simulink model "test_model_2"  (R2017a)
settings: Solver=VariableStepAuto  StartTime=0.0  StopTime=inf  RelTol=1e-3
undefined symbols (not defined in the file): AUV, HydroDyn, kc, Z_delay
libraries: slrealtimeutilitieslib x2, slrealtimeiplib x2, sldrtlib x1, simulink x1
settings Model: Creator=117-11  LastModifiedBy=corsair
settings SFSimCC: SimUseLocalCustomCode=on
settings RTWCC: RTWUseLocalCustomCode=on

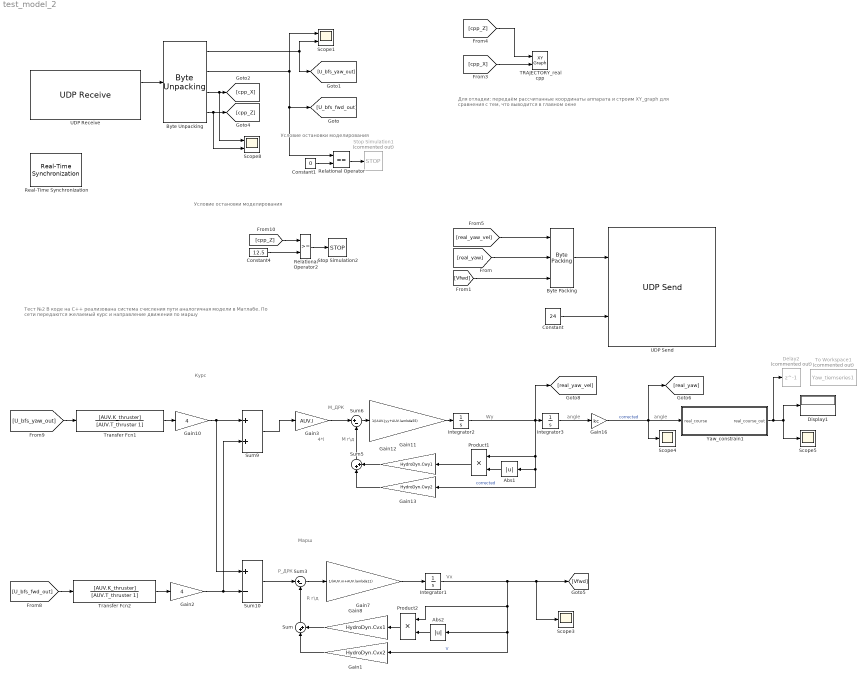
== system test_model_2 ==
  note: Тест №2
      |
      | В коде на С++ реализована система счисления пути аналогичная модели в Матлабе.
      | По сети передаются желаемый курс и направление движения по маршу
  note: Условие остановки моделирования
  note: Для отладки: передаём рассчитанные координаты аппарата и строим XY_graph для сравнения с тем, что выводится в главном окне
  note: Курс
  note: 4*l
  note: Марш
  note: angle
  note: R г\д
  note: Wy
  note: P_ДРК
  note: M_ДРК
  note: M г\д
  note: Vx
  note: angle
  note: Условие остановки моделирования
  Abs1 : Abs
  Abs2 : Abs
  "Byte Packing " : slrealtimeutilitieslib/Byte Packing  MaskPackedDataType=uint8  MaskUnpackedDataTypes={'double', 'double', 'double'}  MaskAlignment=1
  "Byte Unpacking " : slrealtimeutilitieslib/Byte Unpacking  MaskUnpackedDataTypes={'double', 'double', 'double', 'double'}  MaskUnpackedDataSizes={[1], [1], [1], [1]}  MaskAlignment=1
      settings: SourceProductBaseCode=XP
  Constant : Constant  Value=24
  Constant1 : Constant  Value=0
  Constant4 : Constant  Value=12.5
  Delay2 : Delay  Commented=on  DelayLength=1  InitialCondition=180  SampleTime=Z_delay
  Display1 : Display
  Gain1 : Gain  Gain=HydroDyn.Cvx2
  Gain10 : Gain  Gain=4
  Gain11 : Gain  Gain=1/(AUV.Jyy+AUV.lambda55)
  Gain12 : Gain  Gain=HydroDyn.Cwy1
  Gain13 : Gain  Gain=HydroDyn.Cwy2
  Gain16 : Gain  Gain=kc
  Gain2 : Gain  Gain=4
  Gain3 : Gain  Gain=AUV.l
  Gain7 : Gain  Gain=1/(AUV.m+AUV.lambda11)
  Gain8 : Gain  Gain=HydroDyn.Cvx1
  Integrator1 : Integrator  InitialCondition=0.7
  Integrator2 : Integrator
  Integrator3 : Integrator  InitialCondition=3.1416
  Product1 : Product
  Product2 : Product
  Real-Time Synchronization : sldrtlib/Real-Time Synchronization  SampleTime=0.001  MaxMissedTicks=10  ShowMissedTicks=off  YieldWhenWaiting=off
  Relational Operator : RelationalOperator  Operator===  OutDataTypeStr=boolean  RndMeth=Simplest
  Relational Operator2 : RelationalOperator  OutDataTypeStr=boolean  RndMeth=Simplest
  Scope1 : Scope  NumInputPorts=2
  Scope3 : Scope
  Scope4 : Scope
  Scope5 : Scope
  Scope8 : Scope  NumInputPorts=2
  Stop Simulation1 : Stop  Commented=on
  Stop Simulation2 : Stop
  Sum : Sum  Inputs=|++
  Sum10 : Sum  Inputs=+-
  Sum3 : Sum  Inputs=|+-
  Sum5 : Sum  Inputs=|++
  Sum6 : Sum  Inputs=|+-
  Sum9 : Sum
  TRAJECTORY_real cpp : simulink/Sinks/XY Graph  xmin=-15  xmax=15  ymin=-15  ymax=15  st=Z_delay
  To Workspace1 : ToWorkspace  Commented=on  VariableName=Yaw_tiemseries1  SaveFormat=Timeseries  SampleTime=-1
  Transfer Fcn1 : TransferFcn  Numerator=[AUV.K_thruster]  Denominator=[AUV.T_thruster 1]
  Transfer Fcn2 : TransferFcn  Numerator=[AUV.K_thruster]  Denominator=[AUV.T_thruster 1]
  UDP Receive : slrealtimeiplib/UDP Receive  useHostTargetConn=on  ipAddress=10.10.10.15  localPort=13042  rcvWidth=32  rcvFmAny=on  fmAddress=0.0.0.0  rcvMulticast=off  multicastAddress={}  sampleTime=-1
      settings: SourceProductBaseCode=XP
  UDP Send : slrealtimeiplib/UDP Send  useHostTargetConn=on  ipAddress=10.10.10.15  localPort=13043  toAddress=127.0.0.1  toPort=13044  sampleTime=0.001
      settings: SourceProductBaseCode=XP
  Yaw_constrain1 : MATLAB Function  TreatAsAtomicUnit=on
  wires:
  "Byte Unpacking "/1 -> [U_bfs_yaw_out], Scope1/2
  UDP Receive/1 -> "Byte Unpacking "/1
  [real_yaw] -> "Byte Packing "/2
  Constant/1 -> UDP Send/2
  "Byte Packing "/1 -> UDP Send/1
  "Byte Unpacking "/2 -> Relational Operator/1, [U_bfs_fwd_out], Scope1/1
  [Vfwd] -> "Byte Packing "/3
  Relational Operator/1 -> Stop Simulation1/1
  Constant1/1 -> Relational Operator/2
  "Byte Unpacking "/3 -> Scope8/1, [cpp_X]
  "Byte Unpacking "/4 -> Scope8/2, [cpp_Z]
  [cpp_X] -> TRAJECTORY_real cpp/2
  [cpp_Z] -> TRAJECTORY_real cpp/1
  Product2/1 -> Gain8/1
  [U_bfs_fwd_out] -> Transfer Fcn2/1
  Sum3/1 -> Gain7/1
  Gain8/1 -> Sum/2
  Abs1/1 -> Product1/2
  Gain7/1 -> Integrator1/1
  Integrator3/1 -> Gain16/1
  Gain3/1 -> Sum6/1
  Gain1/1 -> Sum/1
  Sum5/1 -> Sum6/2
  Sum6/1 -> Gain11/1
  Gain13/1 -> Sum5/1
  Gain12/1 -> Sum5/2
  Gain11/1 -> Integrator2/1
  Sum/1 -> Sum3/2
  Integrator2/1 -> [real_yaw_vel], Integrator3/1, Abs1/1, Gain13/1, Product1/1  "corrected"
  Transfer Fcn1/1 -> Gain10/1
  Product1/1 -> Gain12/1
  Sum10/1 -> Sum3/1
  [U_bfs_yaw_out] -> Transfer Fcn1/1
  Abs2/1 -> Product2/2
  Gain10/1 -> Sum9/1, Sum10/1
  Gain16/1 -> Scope4/1, [real_yaw], Yaw_constrain1/1(real_course)  "corrected"
  Transfer Fcn2/1 -> Gain2/1
  Gain2/1 -> Sum9/2, Sum10/2
  Sum9/1 -> Gain3/1
  Integrator1/1 -> [Vfwd], Scope3/1, Gain1/1, Abs2/1, Product2/1  "V"
  Yaw_constrain1/1(real_course_out) -> Delay2/1, Scope5/1, Display1/1
  [real_yaw_vel] -> "Byte Packing "/1
  Relational Operator2/1 -> Stop Simulation2/1
  Constant4/1 -> Relational Operator2/2
  [cpp_Z] -> Relational Operator2/1

== matlab function test_model_2/Yaw_constrain1 ==
  data: real_course input; real_course_out output
function real_course_out   = fcn(real_course)

    % Приводим к стандарту
    if real_course < 0
        real_course_out = 360 - abs(real_course);
    elseif real_course >= 360
        real_course_out = real_course - 360;
    else    
        real_course_out = real_course;
    end

end
